simulink model "HybridControllerD3D3"  (Simulink 7.4)
settings: Solver=FixedStepDiscrete  StartTime=0.0  StopTime=inf  FixedStep=samplePeriod  RelTol=1e-3  AbsTol=1e-6
PreLoadFcn:
  | initializeSimulation;
InitFcn:
  | clear('all');
  | initializeSimulation;
undefined symbols (not defined in the file or in its folder): damperA, damperB, damperC, damperCanon, DiscIntNeverNeededParam, flowCanon, forceCanon, frictionA, frictionB, frictionC, gasConstant, HybridCtrlParameters, lengthCanon, massA, massB, massC, massCanon, maxDisplA, maxDisplB, maxDisplC, maxOilVolume, maxVelocA, maxVelocB, maxVelocC, minDisplA, minDisplB, minDisplC, minVelocA, minVelocB, minVelocC, nAct, nAdcU, nDinp, nDout, nDucU, nEncU, precharge, pumpFlow, returnPress, staticForceA, staticForceB, staticForceC, supplyPress, velocCanon, volume, volumeCanon, yieldDisplA, yieldDisplB, yieldDisplC
libraries: simulink x2
(part 1 of 3)
settings Model: Creator=Andreas Schellenberg  LastModifiedBy=Andreas  ExtModeTrigMode=oneshot  ExtModeArmWhenConnect=off  ExtModeAutoUpdateStatusClock=off
settings DataIOCC: SaveOutput=off  SaveTime=off  SignalLoggingName=sigsOut
settings OptimizationCC: EnforceIntegerDowncast=off  InitFltsAndDblsToZero=on
settings DebuggingCC: SaveWithParameterizedLinksMsg=none  CheckSSInitialOutputMsg=off  SolverPrmCheckMsg=none  MultiTaskDSMMsg=warning  MultiTaskCondExecSysMsg=none  StrictBusMsg=None
settings HardwareCC: TargetUnknown=on
settings SFSimCC: SimCustomHeaderCode="#include \"PredictorCorrector.h\""  SimUserSources=PredictorCorrector.c
settings RTWCC: IncludeERTFirstTime=on
settings GRTTargetCC: TargetFcnLib=ansi_tfl_tmw.mat

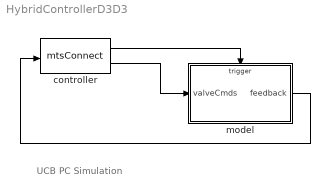
== system HybridControllerD3D3 ==
  note: UCB PC Simulation
  controller : S-Function  FunctionName=mtsConnect  Parameters='127.0.0.1',5002,nUDPInp,nUDPOut  EnableBusSupport=off
  model : Subsystem  TreatAsAtomicUnit=on
  wires:
  model/1(feedback) -> controller/1
  controller/2 -> model/1(valveCmds)
  controller/1 -> model/Trigger

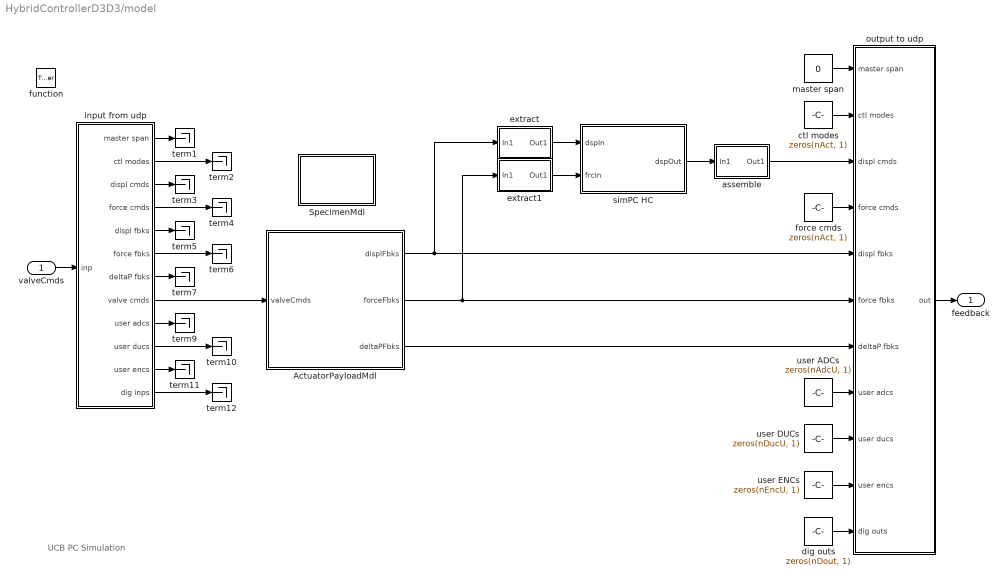
== system HybridControllerD3D3/model ==
  note: UCB PC Simulation
  valveCmds : Inport  OutDataType=sfix(16)  OutScaling=2^0
  function : TriggerPort  TriggerType=function-call
  ActuatorPayloadMdl : Subsystem
  SpecimenMdl : Subsystem
      mask Display: fprintf('Test\nSpecimen');
  assemble : Subsystem  mask(to Actuators){id=1, size=nAct}
      mask prompts: id "Index Vector: id"; size "Vector Size: size"
      mask help: To select to which actuator(s) the signals are going to
      mask Display: disp('Assemble')
  ctl modes : Constant  Value=zeros(nAct, 1)  OutDataType=sfix(16)  OutScaling=2^0
  dig outs : Constant  Value=zeros(nDout, 1)  OutDataTypeMode=uint32  OutDataType=sfix(16)  OutScaling=2^0  OutDataTypeStr=uint32
  extract : Subsystem  mask(from Actuators){id=1, size=nAct}
      mask prompts: id "Index Vector: id"; size "Vector Size: size"
      mask help: To select from which actuator(s) the signals are coming from
      mask Display: disp('Extract')
  extract1 : Subsystem  mask(from Actuators){id=1, size=nAct}
      mask prompts: id "Index Vector: id"; size "Vector Size: size"
      mask help: To select from which actuator(s) the signals are coming from
      mask Display: disp('Extract')
  force cmds : Constant  Value=zeros(nAct, 1)  OutDataType=sfix(16)  OutScaling=2^0
  input from udp : Subsystem
  master span : Constant  Value=0  OutDataType=sfix(16)  OutScaling=2^0
  output to udp : Subsystem
  simPC HC : Subsystem  mask(Hybrid Controller: D3/D3){nAct=1, dtInt=HybridCtrlParameters.dtInt, dtSim=HybridCtrlParameters.dtSim, dtCon=HybridCtrlParameters.dtCon, N=HybridCtrlParameters.N, iDelay=HybridCtrlParameters.iDelay}
      mask prompts: nAct "Number of Actuators: nAct"; dtInt "Integration time step: dtInt"; dtSim "Simulation time step: dtSim"; dtCon "Controller time step: dtCon"; N "Maximum number of substeps: N"; iDelay "Number of delay steps: iDelay"
      mask help: Hybrid Controller using C0-continuous cubic Lagrange interpolation for prediction and correction
      mask Display: disp('simPC Target\nHybrid Controller\n(D3/D3)')
  term{1..7,9..12} (11 alike) : Terminator
  user ADCs : Constant  Value=zeros(nAdcU, 1)  OutDataType=sfix(16)  OutScaling=2^0
  user DUCs : Constant  Value=zeros(nDucU, 1)  OutDataType=sfix(16)  OutScaling=2^0
  user ENCs : Constant  Value=zeros(nEncU, 1)  OutDataType=sfix(16)  OutScaling=2^0
  feedback : Outport  OutDataType=sfix(16)  OutScaling=2^0
  wires:
  input from udp/3(displ cmds) -> term3/1
  input from udp/1(master span) -> term1/1
  input from udp/6(force fbks) -> term6/1
  input from udp/10(user ducs) -> term10/1
  input from udp/12(dig inps) -> term12/1
  input from udp/2(ctl modes) -> term2/1
  input from udp/4(force cmds) -> term4/1
  input from udp/5(displ fbks) -> term5/1
  input from udp/7(deltaP fbks) -> term7/1
  input from udp/9(user adcs) -> term9/1
  input from udp/11(user encs) -> term11/1
  valveCmds/1 -> input from udp/1(inp)
  master span/1 -> output to udp/1(master span)
  ctl modes/1 -> output to udp/2(ctl modes)
  assemble/1(Out1) -> output to udp/3(displ cmds)
  force cmds/1 -> output to udp/4(force cmds)
  user ADCs/1 -> output to udp/8(user adcs)
  user DUCs/1 -> output to udp/9(user ducs)
  user ENCs/1 -> output to udp/10(user encs)
  dig outs/1 -> output to udp/11(dig outs)
  output to udp/1(out) -> feedback/1
  ActuatorPayloadMdl/1(displFbks) -> output to udp/5(displ fbks), extract/1(In1)
  ActuatorPayloadMdl/2(forceFbks) -> output to udp/6(force fbks), extract1/1(In1)
  ActuatorPayloadMdl/3(deltaPFbks) -> output to udp/7(deltaP fbks)
  input from udp/8(valve cmds) -> ActuatorPayloadMdl/1(valveCmds)
  extract1/1(Out1) -> simPC HC/2(frcIn)
  extract/1(Out1) -> simPC HC/1(dspIn)
  simPC HC/1(dspOut) -> assemble/1(In1)

== system HybridControllerD3D3/model/ActuatorPayloadMdl ==
  valveCmds : Inport  OutDataType=sfix(16)  OutScaling=2^0
  Demux : Demux  Outputs=nAct
  Mux : Mux  Inputs=nAct
  Mux1 : Mux  Inputs=nAct
  Mux2 : Mux  Inputs=nAct
  Sum : Sum  Inputs=++++++++  OutDataType=sfix(16)  OutScaling=2^0  SaturateOnIntegerOverflow=on
  accumulators : Subsystem
  dynamic long channel #1 : Subsystem
  dynamic long channel #2 : Subsystem
  dynamic short channel #1 : Subsystem
  dynamic short channel #2 : Subsystem
  static channel #1 : Subsystem
  static channel #2 : Subsystem
  static channel #3 : Subsystem
  static channel #4 : Subsystem
  displFbks : Outport  OutDataType=sfix(16)  OutScaling=2^0
  forceFbks : Outport  Port=2  OutDataType=sfix(16)  OutScaling=2^0
  deltaPFbks : Outport  Port=3  OutDataType=sfix(16)  OutScaling=2^0
  wires:
  Demux/1 -> dynamic short channel #1/1(valve cmd)
  Demux/3 -> dynamic long channel #1/1(valve cmd)
  Demux/2 -> dynamic short channel #2/1(valve cmd)
  dynamic short channel #1/4(flow) -> Sum/1
  dynamic short channel #2/4(flow) -> Sum/2
  dynamic long channel #1/4(flow) -> Sum/3
  Sum/1 -> accumulators/1(flow)
  Demux/4 -> dynamic long channel #2/1(valve cmd)
  Demux/5 -> static channel #1/1(valve cmd)
  Demux/6 -> static channel #2/1(valve cmd)
  Demux/7 -> static channel #3/1(valve cmd)
  Demux/8 -> static channel #4/1(valve cmd)
  dynamic long channel #2/4(flow) -> Sum/4
  static channel #1/4(flow) -> Sum/5
  static channel #2/4(flow) -> Sum/6
  static channel #3/4(flow) -> Sum/7
  static channel #4/4(flow) -> Sum/8
  accumulators/1(press) -> static channel #4/2(spl press), static channel #3/2(spl press), static channel #2/2(spl press), static channel #1/2(spl press), dynamic long channel #2/2(spl press), dynamic long channel #1/2(spl press), dynamic short channel #2/2(spl press), dynamic short channel #1/2(spl press)
  dynamic short channel #1/1(displ) -> Mux/1
  dynamic short channel #2/1(displ) -> Mux/2
  dynamic long channel #1/1(displ) -> Mux/3
  dynamic long channel #2/1(displ) -> Mux/4
  static channel #1/1(displ) -> Mux/5
  static channel #2/1(displ) -> Mux/6
  static channel #3/1(displ) -> Mux/7
  static channel #4/1(displ) -> Mux/8
  dynamic short channel #1/2(force) -> Mux1/1
  dynamic short channel #2/2(force) -> Mux1/2
  dynamic long channel #1/2(force) -> Mux1/3
  dynamic long channel #2/2(force) -> Mux1/4
  static channel #1/2(force) -> Mux1/5
  static channel #2/2(force) -> Mux1/6
  static channel #3/2(force) -> Mux1/7
  static channel #4/2(force) -> Mux1/8
  dynamic short channel #1/3(dpforce) -> Mux2/1
  dynamic short channel #2/3(dpforce) -> Mux2/2
  dynamic long channel #1/3(dpforce) -> Mux2/3
  dynamic long channel #2/3(dpforce) -> Mux2/4
  static channel #1/3(dpforce) -> Mux2/5
  static channel #2/3(dpforce) -> Mux2/6
  static channel #3/3(dpforce) -> Mux2/7
  static channel #4/3(dpforce) -> Mux2/8
  valveCmds/1 -> Demux/1
  Mux/1 -> displFbks/1
  Mux1/1 -> forceFbks/1
  Mux2/1 -> deltaPFbks/1

== system HybridControllerD3D3/model/SpecimenMdl ==
  Scope3 : Scope
      settings: TimeRange=250  YMin=-2  YMax=2  SaveName=ScopeData2
  Specimen #1 : S-Function  FunctionName=SFun_SimFEAdapter  Parameters=ipAddr,ipPort,dataSize  EnableBusSupport=off  mask(GenericClient Element){ipAddr=127.0.0.1, ipPort=44000, dataSize=256}
      mask prompts: ipAddr "IP Address of Adapter Element"; ipPort "IP Port Number of Adapter Element"; dataSize "Size of Data Arrays"
      mask Display: disp('SimFE\nAdapter');
  Terminator : Terminator
  assemble1 : Subsystem  mask(to Actuators){id=1, size=nAct}
      mask prompts: id "Index Vector: id"; size "Vector Size: size"
      mask help: To select to which actuator(s) the signals are going to
      mask Display: disp('Assemble')
  assemble2 : Subsystem  mask(to Actuators){id=1, size=nAct}
      mask prompts: id "Index Vector: id"; size "Vector Size: size"
      mask help: To select to which actuator(s) the signals are going to
      mask Display: disp('Assemble')
  extract2 : Subsystem  mask(from Actuators){id=1, size=nAct}
      mask prompts: id "Index Vector: id"; size "Vector Size: size"
      mask help: To select from which actuator(s) the signals are coming from
      mask Display: disp('Extract')
  from Actuators : Subsystem
  to LoadCells : Subsystem
  wires:
  from Actuators/1(ctrlDisp) -> extract2/1(In1)
  extract2/1(Out1) -> Specimen #1/1
  Specimen #1/1 -> assemble2/1(In1)
  Specimen #1/2 -> assemble1/1(In1), Scope3/1
  assemble2/1(Out1) -> Terminator/1
  assemble1/1(Out1) -> to LoadCells/1(daqForce)

== system HybridControllerD3D3/model/assemble ==
  In1 : Inport  OutDataType=sfix(16)  OutScaling=2^0
  Assignment : Assignment  OutputInitialize=Specify size for each dimension in table  IndexOptions=Index vector (port)  Indices=1  OutputSizes=nAct
  Constant : Constant  Value=id  OutDataType=sfix(16)  OutScaling=2^0
  Out1 : Outport  OutDataType=sfix(16)  OutScaling=2^0
  wires:
  Constant/1 -> Assignment/2
  Assignment/1 -> Out1/1
  In1/1 -> Assignment/1

== system HybridControllerD3D3/model/extract ==
  In1 : Inport  OutDataType=sfix(16)  OutScaling=2^0
  Selector : Selector  InputPortWidth=size  IndexOptions=Index vector (dialog)  Indices=id  OutputSizes=1
  Out1 : Outport  OutDataType=sfix(16)  OutScaling=2^0
  wires:
  Selector/1 -> Out1/1
  In1/1 -> Selector/1

== system HybridControllerD3D3/model/extract1 ==
  In1 : Inport  OutDataType=sfix(16)  OutScaling=2^0
  Selector : Selector  InputPortWidth=size  IndexOptions=Index vector (dialog)  Indices=id  OutputSizes=1
  Out1 : Outport  OutDataType=sfix(16)  OutScaling=2^0
  wires:
  Selector/1 -> Out1/1
  In1/1 -> Selector/1

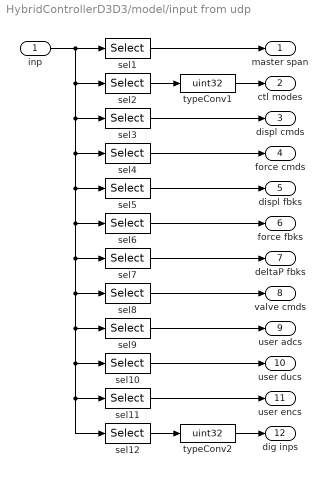
== system HybridControllerD3D3/model/input from udp ==
  inp : Inport  OutDataType=sfix(16)  OutScaling=2^0
  sel1 : Selector  InputPortWidth=nUDPOut  IndexOptions=Index vector (dialog)  Indices=[0]+1  OutputSizes=1
  sel10 : Selector  InputPortWidth=nUDPOut  IndexOptions=Index vector (dialog)  Indices=[1:nDucU]+1+7*nAct+nAdcU  OutputSizes=1
  sel11 : Selector  InputPortWidth=nUDPOut  IndexOptions=Index vector (dialog)  Indices=[1:nEncU]+1+7*nAct+nAdcU+nDucU  OutputSizes=1
  sel12 : Selector  InputPortWidth=nUDPOut  IndexOptions=Index vector (dialog)  Indices=[1:nDinp]+1+7*nAct+nAdcU+nDucU+nEncU  OutputSizes=1
  sel2 : Selector  InputPortWidth=nUDPOut  IndexOptions=Index vector (dialog)  Indices=[1:nAct]+1+0*nAct  OutputSizes=1
  sel3 : Selector  InputPortWidth=nUDPOut  IndexOptions=Index vector (dialog)  Indices=[1:nAct]+1+1*nAct  OutputSizes=1
  sel4 : Selector  InputPortWidth=nUDPOut  IndexOptions=Index vector (dialog)  Indices=[1:nAct]+1+2*nAct  OutputSizes=1
  sel5 : Selector  InputPortWidth=nUDPOut  IndexOptions=Index vector (dialog)  Indices=[1:nAct]+1+3*nAct  OutputSizes=1
  sel6 : Selector  InputPortWidth=nUDPOut  IndexOptions=Index vector (dialog)  Indices=[1:nAct]+1+4*nAct  OutputSizes=1
  sel7 : Selector  InputPortWidth=nUDPOut  IndexOptions=Index vector (dialog)  Indices=[1:nAct]+1+5*nAct  OutputSizes=1
  sel8 : Selector  InputPortWidth=nUDPOut  IndexOptions=Index vector (dialog)  Indices=[1:nAct]+1+6*nAct  OutputSizes=1
  sel9 : Selector  InputPortWidth=nUDPOut  IndexOptions=Index vector (dialog)  Indices=[1:nAdcU]+1+7*nAct  OutputSizes=1
  typeConv1 : DataTypeConversion  OutDataTypeMode=uint32  OutDataType=sfix(16)  OutScaling=2^0  OutDataTypeStr=uint32  SaturateOnIntegerOverflow=on  RndMeth=Zero
  typeConv2 : DataTypeConversion  OutDataTypeMode=uint32  OutDataType=sfix(16)  OutScaling=2^0  OutDataTypeStr=uint32  SaturateOnIntegerOverflow=on  RndMeth=Zero
  master span : Outport  OutDataType=sfix(16)  OutScaling=2^0
  ctl modes : Outport  Port=2  OutDataType=sfix(16)  OutScaling=2^0
  displ cmds : Outport  Port=3  OutDataType=sfix(16)  OutScaling=2^0
  force cmds : Outport  Port=4  OutDataType=sfix(16)  OutScaling=2^0
  displ fbks : Outport  Port=5  OutDataType=sfix(16)  OutScaling=2^0
  force fbks : Outport  Port=6  OutDataType=sfix(16)  OutScaling=2^0
  deltaP fbks : Outport  Port=7  OutDataType=sfix(16)  OutScaling=2^0
  valve cmds : Outport  Port=8  OutDataType=sfix(16)  OutScaling=2^0
  user adcs : Outport  Port=9  OutDataType=sfix(16)  OutScaling=2^0
  user ducs : Outport  Port=10  OutDataType=sfix(16)  OutScaling=2^0
  user encs : Outport  Port=11  OutDataType=sfix(16)  OutScaling=2^0
  dig inps : Outport  Port=12  OutDataType=sfix(16)  OutScaling=2^0
  wires:
  sel1/1 -> master span/1
  sel2/1 -> typeConv1/1
  sel3/1 -> displ cmds/1
  sel4/1 -> force cmds/1
  sel5/1 -> displ fbks/1
  sel6/1 -> force fbks/1
  sel7/1 -> deltaP fbks/1
  sel8/1 -> valve cmds/1
  sel9/1 -> user adcs/1
  sel10/1 -> user ducs/1
  sel11/1 -> user encs/1
  sel12/1 -> typeConv2/1
  inp/1 -> sel1/1, sel2/1, sel3/1, sel11/1, sel12/1, sel10/1, sel9/1, sel8/1, sel7/1, sel6/1, sel5/1, sel4/1
  typeConv1/1 -> ctl modes/1
  typeConv2/1 -> dig inps/1

== system HybridControllerD3D3/model/output to udp ==
  master span : Inport  OutDataType=sfix(16)  OutScaling=2^0
  ctl modes : Inport  Port=2  OutDataType=sfix(16)  OutScaling=2^0
  displ cmds : Inport  Port=3  OutDataType=sfix(16)  OutScaling=2^0
  force cmds : Inport  Port=4  OutDataType=sfix(16)  OutScaling=2^0
  displ fbks : Inport  Port=5  OutDataType=sfix(16)  OutScaling=2^0
  force fbks : Inport  Port=6  OutDataType=sfix(16)  OutScaling=2^0
  deltaP fbks : Inport  Port=7  OutDataType=sfix(16)  OutScaling=2^0
  user adcs : Inport  Port=8  OutDataType=sfix(16)  OutScaling=2^0
  user ducs : Inport  Port=9  OutDataType=sfix(16)  OutScaling=2^0
  user encs : Inport  Port=10  OutDataType=sfix(16)  OutScaling=2^0
  dig outs : Inport  Port=11  OutDataType=sfix(16)  OutScaling=2^0
  Mux : Mux  Inputs=11
  typeConv1 : DataTypeConversion  OutDataTypeMode=double  OutDataType=sfix(16)  OutScaling=2^0  OutDataTypeStr=double  SaturateOnIntegerOverflow=on  RndMeth=Zero
  typeConv2 : DataTypeConversion  OutDataTypeMode=double  OutDataType=sfix(16)  OutScaling=2^0  OutDataTypeStr=double  SaturateOnIntegerOverflow=on  RndMeth=Zero
  out : Outport  OutDataType=sfix(16)  OutScaling=2^0
  wires:
  typeConv2/1 -> Mux/11
  dig outs/1 -> typeConv2/1
  user encs/1 -> Mux/10
  user ducs/1 -> Mux/9
  user adcs/1 -> Mux/8
  deltaP fbks/1 -> Mux/7
  force fbks/1 -> Mux/6
  displ fbks/1 -> Mux/5
  force cmds/1 -> Mux/4
  master span/1 -> Mux/1
  displ cmds/1 -> Mux/3
  ctl modes/1 -> typeConv1/1
  Mux/1 -> out/1
  typeConv1/1 -> Mux/2

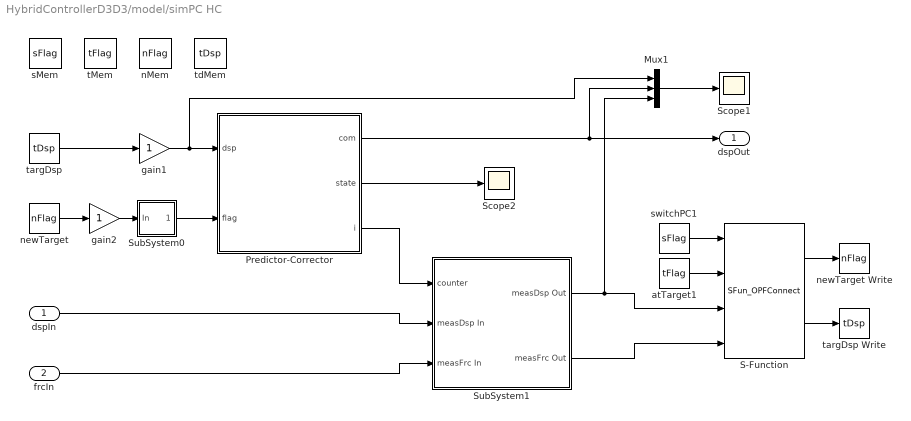
== system HybridControllerD3D3/model/simPC HC ==
  dspIn : Inport  OutDataType=sfix(16)  OutScaling=2^0
  frcIn : Inport  Port=2  OutDataType=sfix(16)  OutScaling=2^0
  Mux1 : Mux  Inputs=3
  Predictor-Corrector : Stateflow chart
  S-Function : S-Function  FunctionName=SFun_OPFConnect  Parameters=ipPort  EnableBusSupport=off  mask(OpenFresco Connect){ipPort=8090}
      mask prompts: ipPort "IP Port Number of Server"
      mask Display: disp('OpenFresco\nConnect');
  Scope1 : Scope
      settings: TimeRange=250  YMin=-2  YMax=2.5  SaveName=ScopeData3
  Scope2 : Scope
      settings: TimeRange=250  YMin=0  YMax=2  SaveName=ScopeData2
  SubSystem0 : Subsystem
  SubSystem1 : Subsystem
  atTarget1 : DataStoreRead  DataStoreName=tFlag  SampleTime=-1
  gain1 : Gain  ParameterDataType=sfix(16)  ParameterScaling=2^0  OutDataType=sfix(16)  OutScaling=2^0
  gain2 : Gain  ParameterDataType=sfix(16)  ParameterScaling=2^0  OutDataType=sfix(16)  OutScaling=2^0
  nMem : DataStoreMemory  DataStoreName=nFlag  DataType=double  OutDataType=sfix(16)  OutScaling=2^0  OutDataTypeStr=double
  newTarget : DataStoreRead  DataStoreName=nFlag  SampleTime=-1
  newTarget Write : DataStoreWrite  DataStoreName=nFlag  SampleTime=-1
  sMem : DataStoreMemory  DataStoreName=sFlag  DataType=double  OutDataType=sfix(16)  OutScaling=2^0  OutDataTypeStr=double
  switchPC1 : DataStoreRead  DataStoreName=sFlag  SampleTime=-1
  tMem : DataStoreMemory  DataStoreName=tFlag  DataType=double  OutDataType=sfix(16)  OutScaling=2^0  OutDataTypeStr=double
  targDsp : DataStoreRead  DataStoreName=tDsp  SampleTime=-1
  targDsp Write : DataStoreWrite  DataStoreName=tDsp  SampleTime=-1
  tdMem : DataStoreMemory  DataStoreName=tDsp  DataType=double  OutDataType=sfix(16)  OutScaling=2^0  OutDataTypeStr=double
  dspOut : Outport  OutDataType=sfix(16)  OutScaling=2^0
  wires:
  frcIn/1 -> SubSystem1/3(measFrc In)
  dspIn/1 -> SubSystem1/2(measDsp In)
  SubSystem1/2(measFrc Out) -> S-Function/4
  SubSystem1/1(measDsp Out) -> Mux1/3, S-Function/3
  Predictor-Corrector/3(i) -> SubSystem1/1(counter)
  Predictor-Corrector/2(state) -> Scope2/1
  Predictor-Corrector/1(com) -> dspOut/1, Mux1/2
  SubSystem0/1(Out) -> Predictor-Corrector/2(flag)
  newTarget/1 -> gain2/1
  gain2/1 -> SubSystem0/1(In)
  targDsp/1 -> gain1/1
  gain1/1 -> Predictor-Corrector/1(dsp), Mux1/1
  Mux1/1 -> Scope1/1
  switchPC1/1 -> S-Function/1
  atTarget1/1 -> S-Function/2
  S-Function/1 -> newTarget Write/1
  S-Function/2 -> targDsp Write/1

== system HybridControllerD3D3/model/ActuatorPayloadMdl/accumulators ==
  flow : Inport  OutDataType=sfix(16)  OutScaling=2^0
  Sum : Sum  Inputs=+-|  OutDataType=sfix(16)  OutScaling=2^0  SaturateOnIntegerOverflow=on  InputSameDT=on  OutDataTypeStr=Inherit: Same as first input
  Sum1 : Sum  Inputs=+-|  OutDataType=sfix(16)  OutScaling=2^0  SaturateOnIntegerOverflow=on  InputSameDT=on  OutDataTypeStr=Inherit: Same as first input
  bottle volume : Constant  Value=volume*volumeCanon  OutDataType=sfix(16)  OutScaling=2^0
  flowCanon : Gain  Gain=flowCanon  ParameterDataType=sfix(16)  ParameterScaling=2^0  OutDataType=sfix(16)  OutScaling=2^0  SaturateOnIntegerOverflow=on  OutDataTypeStr=Inherit: Same as input  ParamDataTypeStr=Inherit: Same as input
  gas constant : Constant  Value=gasConstant  OutDataType=sfix(16)  OutScaling=2^0
  initial condition : UnitDelay  X0=supplyPress  SampleTime=-1
  integrator : DiscreteIntegrator  InitialCondition=maxOilVolume*volumeCanon  SampleTime=-1  OutDataType=sfix(16)  OutScaling=2^0  LimitOutput=on  UpperSaturationLimit=maxOilVolume*volumeCanon  LowerSaturationLimit=0  ICPrevOutput=DiscIntNeverNeededParam  ICPrevScaledInput=DiscIntNeverNeededParam
  power : Math  Operator=pow  OutDataType=sfix(16)  OutScaling=2^0  SaturateOnIntegerOverflow=on
  precharge : Gain  Gain=precharge  ParameterDataType=sfix(16)  ParameterScaling=2^0  OutDataType=sfix(16)  OutScaling=2^0  SaturateOnIntegerOverflow=on  OutDataTypeStr=Inherit: Same as input  ParamDataTypeStr=Inherit: Same as input
  pump flow : Constant  Value=pumpFlow  OutDataType=sfix(16)  OutScaling=2^0
  quotient : Product  Inputs=*/  OutDataType=sfix(16)  OutScaling=2^0  SaturateOnIntegerOverflow=on  InputSameDT=on  OutDataTypeStr=Inherit: Same as first input
  press : Outport  OutDataType=sfix(16)  OutScaling=2^0
  wires:
  initial condition/1 -> press/1
  flowCanon/1 -> integrator/1
  flow/1 -> Sum/2
  integrator/1 -> Sum1/2  "current oil volume"
  quotient/1 -> power/1
  Sum1/1 -> quotient/2  "current gas volume"
  precharge/1 -> initial condition/1
  power/1 -> precharge/1
  gas constant/1 -> power/2
  bottle volume/1 -> quotient/1, Sum1/1
  Sum/1 -> flowCanon/1
  pump flow/1 -> Sum/1

== system HybridControllerD3D3/model/ActuatorPayloadMdl/dynamic long channel #1 ==
  valve cmd : Inport  OutDataType=sfix(16)  OutScaling=2^0
  spl press : Inport  Port=2  OutDataType=sfix(16)  OutScaling=2^0
  actuator/valve  model : Subsystem
      mask Type: Inverse Actuator
  payload : Subsystem
  return pressure : Constant  Value=returnPress  OutDataType=sfix(16)  OutScaling=2^0
  displ : Outport  OutDataType=sfix(16)  OutScaling=2^0
  force : Outport  Port=2  OutDataType=sfix(16)  OutScaling=2^0
  dpforce : Outport  Port=3  OutDataType=sfix(16)  OutScaling=2^0
  flow : Outport  Port=4  OutDataType=sfix(16)  OutScaling=2^0
  wires:
  payload/2(veloc) -> actuator/valve  model/3(veloc)
  payload/1(displ) -> displ/1, actuator/valve  model/2(displ)
  valve cmd/1 -> actuator/valve  model/1(cmd)
  return pressure/1 -> actuator/valve  model/5(rtn press)
  spl press/1 -> actuator/valve  model/4(spl press)
  actuator/valve  model/2(flow) -> flow/1
  actuator/valve  model/1(force) -> force/1, dpforce/1, payload/1(force)

== system HybridControllerD3D3/model/ActuatorPayloadMdl/dynamic long channel #2 ==
  valve cmd : Inport  OutDataType=sfix(16)  OutScaling=2^0
  spl press : Inport  Port=2  OutDataType=sfix(16)  OutScaling=2^0
  actuator/valve  model : Subsystem
      mask Type: Inverse Actuator
  payload : Subsystem
  return pressure : Constant  Value=returnPress  OutDataType=sfix(16)  OutScaling=2^0
  displ : Outport  OutDataType=sfix(16)  OutScaling=2^0
  force : Outport  Port=2  OutDataType=sfix(16)  OutScaling=2^0
  dpforce : Outport  Port=3  OutDataType=sfix(16)  OutScaling=2^0
  flow : Outport  Port=4  OutDataType=sfix(16)  OutScaling=2^0
  wires:
  actuator/valve  model/1(force) -> dpforce/1, force/1, payload/1(force)
  actuator/valve  model/2(flow) -> flow/1
  spl press/1 -> actuator/valve  model/4(spl press)
  return pressure/1 -> actuator/valve  model/5(rtn press)
  valve cmd/1 -> actuator/valve  model/1(cmd)
  payload/1(displ) -> actuator/valve  model/2(displ), displ/1
  payload/2(veloc) -> actuator/valve  model/3(veloc)

== system HybridControllerD3D3/model/ActuatorPayloadMdl/dynamic short channel #1 ==
  valve cmd : Inport  OutDataType=sfix(16)  OutScaling=2^0
  spl press : Inport  Port=2  OutDataType=sfix(16)  OutScaling=2^0
  actuator/valve  model : Subsystem
      mask Type: Inverse Actuator
  payload : Subsystem
  return pressure : Constant  Value=returnPress  OutDataType=sfix(16)  OutScaling=2^0
  displ : Outport  OutDataType=sfix(16)  OutScaling=2^0
  force : Outport  Port=2  OutDataType=sfix(16)  OutScaling=2^0
  dpforce : Outport  Port=3  OutDataType=sfix(16)  OutScaling=2^0
  flow : Outport  Port=4  OutDataType=sfix(16)  OutScaling=2^0
  wires:
  actuator/valve  model/1(force) -> dpforce/1, force/1, payload/1(force)
  actuator/valve  model/2(flow) -> flow/1
  spl press/1 -> actuator/valve  model/4(spl press)
  return pressure/1 -> actuator/valve  model/5(rtn press)
  valve cmd/1 -> actuator/valve  model/1(cmd)
  payload/1(displ) -> actuator/valve  model/2(displ), displ/1
  payload/2(veloc) -> actuator/valve  model/3(veloc)

== system HybridControllerD3D3/model/ActuatorPayloadMdl/dynamic short channel #2 ==
  valve cmd : Inport  OutDataType=sfix(16)  OutScaling=2^0
  spl press : Inport  Port=2  OutDataType=sfix(16)  OutScaling=2^0
  actuator/valve  model : Subsystem
      mask Type: Inverse Actuator
  payload : Subsystem
  return pressure : Constant  Value=returnPress  OutDataType=sfix(16)  OutScaling=2^0
  displ : Outport  OutDataType=sfix(16)  OutScaling=2^0
  force : Outport  Port=2  OutDataType=sfix(16)  OutScaling=2^0
  dpforce : Outport  Port=3  OutDataType=sfix(16)  OutScaling=2^0
  flow : Outport  Port=4  OutDataType=sfix(16)  OutScaling=2^0
  wires:
  actuator/valve  model/1(force) -> dpforce/1, force/1, payload/1(force)
  actuator/valve  model/2(flow) -> flow/1
  spl press/1 -> actuator/valve  model/4(spl press)
  return pressure/1 -> actuator/valve  model/5(rtn press)
  valve cmd/1 -> actuator/valve  model/1(cmd)
  payload/1(displ) -> actuator/valve  model/2(displ), displ/1
  payload/2(veloc) -> actuator/valve  model/3(veloc)

== system HybridControllerD3D3/model/ActuatorPayloadMdl/static channel #1 ==
  valve cmd : Inport  OutDataType=sfix(16)  OutScaling=2^0
  spl press : Inport  Port=2  OutDataType=sfix(16)  OutScaling=2^0
  actuator/valve  model : Subsystem
      mask Type: Inverse Actuator
  payload : Subsystem
  return pressure : Constant  Value=returnPress  OutDataType=sfix(16)  OutScaling=2^0
  displ : Outport  OutDataType=sfix(16)  OutScaling=2^0
  force : Outport  Port=2  OutDataType=sfix(16)  OutScaling=2^0
  dpforce : Outport  Port=3  OutDataType=sfix(16)  OutScaling=2^0
  flow : Outport  Port=4  OutDataType=sfix(16)  OutScaling=2^0
  wires:
  payload/2(veloc) -> actuator/valve  model/3(veloc)
  payload/1(displ) -> displ/1, actuator/valve  model/2(displ)
  valve cmd/1 -> actuator/valve  model/1(cmd)
  return pressure/1 -> actuator/valve  model/5(rtn press)
  spl press/1 -> actuator/valve  model/4(spl press)
  actuator/valve  model/2(flow) -> flow/1
  actuator/valve  model/1(force) -> force/1, dpforce/1, payload/1(force)

== system HybridControllerD3D3/model/ActuatorPayloadMdl/static channel #2 ==
  valve cmd : Inport  OutDataType=sfix(16)  OutScaling=2^0
  spl press : Inport  Port=2  OutDataType=sfix(16)  OutScaling=2^0
  actuator/valve  model : Subsystem
      mask Type: Inverse Actuator
  payload : Subsystem
  return pressure : Constant  Value=returnPress  OutDataType=sfix(16)  OutScaling=2^0
  displ : Outport  OutDataType=sfix(16)  OutScaling=2^0
  force : Outport  Port=2  OutDataType=sfix(16)  OutScaling=2^0
  dpforce : Outport  Port=3  OutDataType=sfix(16)  OutScaling=2^0
  flow : Outport  Port=4  OutDataType=sfix(16)  OutScaling=2^0
  wires:
  actuator/valve  model/1(force) -> dpforce/1, force/1, payload/1(force)
  actuator/valve  model/2(flow) -> flow/1
  spl press/1 -> actuator/valve  model/4(spl press)
  return pressure/1 -> actuator/valve  model/5(rtn press)
  valve cmd/1 -> actuator/valve  model/1(cmd)
  payload/1(displ) -> actuator/valve  model/2(displ), displ/1
  payload/2(veloc) -> actuator/valve  model/3(veloc)

== system HybridControllerD3D3/model/ActuatorPayloadMdl/static channel #3 ==
  valve cmd : Inport  OutDataType=sfix(16)  OutScaling=2^0
  spl press : Inport  Port=2  OutDataType=sfix(16)  OutScaling=2^0
  actuator/valve  model : Subsystem
      mask Type: Inverse Actuator
  payload : Subsystem
  return pressure : Constant  Value=returnPress  OutDataType=sfix(16)  OutScaling=2^0
  displ : Outport  OutDataType=sfix(16)  OutScaling=2^0
  force : Outport  Port=2  OutDataType=sfix(16)  OutScaling=2^0
  dpforce : Outport  Port=3  OutDataType=sfix(16)  OutScaling=2^0
  flow : Outport  Port=4  OutDataType=sfix(16)  OutScaling=2^0
  wires:
  payload/2(veloc) -> actuator/valve  model/3(veloc)
  payload/1(displ) -> displ/1, actuator/valve  model/2(displ)
  valve cmd/1 -> actuator/valve  model/1(cmd)
  return pressure/1 -> actuator/valve  model/5(rtn press)
  spl press/1 -> actuator/valve  model/4(spl press)
  actuator/valve  model/2(flow) -> flow/1
  actuator/valve  model/1(force) -> force/1, dpforce/1, payload/1(force)

== system HybridControllerD3D3/model/ActuatorPayloadMdl/static channel #4 ==
  valve cmd : Inport  OutDataType=sfix(16)  OutScaling=2^0
  spl press : Inport  Port=2  OutDataType=sfix(16)  OutScaling=2^0
  actuator/valve  model : Subsystem
      mask Type: Inverse Actuator
  payload : Subsystem
  return pressure : Constant  Value=returnPress  OutDataType=sfix(16)  OutScaling=2^0
  displ : Outport  OutDataType=sfix(16)  OutScaling=2^0
  force : Outport  Port=2  OutDataType=sfix(16)  OutScaling=2^0
  dpforce : Outport  Port=3  OutDataType=sfix(16)  OutScaling=2^0
  flow : Outport  Port=4  OutDataType=sfix(16)  OutScaling=2^0
  wires:
  actuator/valve  model/1(force) -> dpforce/1, force/1, payload/1(force)
  actuator/valve  model/2(flow) -> flow/1
  spl press/1 -> actuator/valve  model/4(spl press)
  return pressure/1 -> actuator/valve  model/5(rtn press)
  valve cmd/1 -> actuator/valve  model/1(cmd)
  payload/1(displ) -> actuator/valve  model/2(displ), displ/1
  payload/2(veloc) -> actuator/valve  model/3(veloc)

== system HybridControllerD3D3/model/SpecimenMdl/assemble1 ==
  In1 : Inport  OutDataType=sfix(16)  OutScaling=2^0
  Assignment : Assignment  OutputInitialize=Specify size for each dimension in table  IndexOptions=Index vector (port)  Indices=1  OutputSizes=nAct
  Constant : Constant  Value=id  OutDataType=sfix(16)  OutScaling=2^0
  Out1 : Outport  OutDataType=sfix(16)  OutScaling=2^0
  wires:
  Constant/1 -> Assignment/2
  Assignment/1 -> Out1/1
  In1/1 -> Assignment/1

== system HybridControllerD3D3/model/SpecimenMdl/assemble2 ==
  In1 : Inport  OutDataType=sfix(16)  OutScaling=2^0
  Assignment : Assignment  OutputInitialize=Specify size for each dimension in table  IndexOptions=Index vector (port)  Indices=1  OutputSizes=nAct
  Constant : Constant  Value=id  OutDataType=sfix(16)  OutScaling=2^0
  Out1 : Outport  OutDataType=sfix(16)  OutScaling=2^0
  wires:
  Constant/1 -> Assignment/2
  Assignment/1 -> Out1/1
  In1/1 -> Assignment/1

== system HybridControllerD3D3/model/SpecimenMdl/extract2 ==
  In1 : Inport  OutDataType=sfix(16)  OutScaling=2^0
  Selector : Selector  InputPortWidth=size  IndexOptions=Index vector (dialog)  Indices=id  OutputSizes=1
  Out1 : Outport  OutDataType=sfix(16)  OutScaling=2^0
  wires:
  Selector/1 -> Out1/1
  In1/1 -> Selector/1

== system HybridControllerD3D3/model/SpecimenMdl/from Actuators ==
  Bus Creator : BusCreator  Inputs=8
  ctrlDisp : Outport
  wires:
  [ch1a] -> Bus Creator/1
  [ch2a] -> Bus Creator/2
  [ch3a] -> Bus Creator/3
  [ch4a] -> Bus Creator/4
  [ch5a] -> Bus Creator/5
  [ch6a] -> Bus Creator/6
  [ch7a] -> Bus Creator/7
  [ch8a] -> Bus Creator/8
  Bus Creator/1 -> ctrlDisp/1

== system HybridControllerD3D3/model/SpecimenMdl/to LoadCells ==
  daqForce : Inport
  Demux : Demux  Outputs=8
  tag scope: ch1b=global, ch2b=global, ch3b=global, ch4b=global, ch5b=global, ch6b=global, ch7b=global, ch8b=global
  wires:
  Demux/1 -> [ch1b]
  Demux/2 -> [ch2b]
  Demux/3 -> [ch3b]
  Demux/4 -> [ch4b]
  Demux/5 -> [ch5b]
  Demux/6 -> [ch6b]
  Demux/7 -> [ch7b]
  Demux/8 -> [ch8b]
  daqForce/1 -> Demux/1

== system HybridControllerD3D3/model/simPC HC/SubSystem0 ==
  In : Inport  OutDataType=sfix(16)  OutScaling=2^0
  Detect Fall Nonpositive : simulink/Logic and Bit Operations/Detect Fall Nonpositive  SystemSampleTime=-1  vinit=0
  Detect Rise Positive : simulink/Logic and Bit Operations/Detect Rise Positive  SystemSampleTime=-1  vinit=0
  If Action Subsystem0 : Subsystem  TreatAsAtomicUnit=on
  If Action Subsystem1 : Subsystem  TreatAsAtomicUnit=on
  If0 : If  IfExpression=u1 == 1  ShowElse=off
  If1 : If  IfExpression=u1 == 1  ShowElse=off
  Mux1 : Mux  Inputs=3
  Scope3 : Scope
      settings: TimeRange=250  YMin=0  YMax=1
  atTarget1 : DataStoreRead  DataStoreName=tFlag  SampleTime=-1
  switchPC1 : DataStoreRead  DataStoreName=sFlag  SampleTime=-1
  typeConv : DataTypeConversion  OutDataTypeMode=double  OutDataType=sfix(16)  OutScaling=2^0  OutDataTypeStr=double  SaturateOnIntegerOverflow=on  RndMeth=Zero
  Out : Outport  OutDataType=sfix(16)  OutScaling=2^0
  wires:
  In/1 -> Detect Rise Positive/1, Detect Fall Nonpositive/1, Mux1/1
  Detect Rise Positive/1 -> If0/1, typeConv/1
  Detect Fall Nonpositive/1 -> If1/1
  If1/1 -> If Action Subsystem1/Action
  If0/1 -> If Action Subsystem0/Action
  typeConv/1 -> Out/1
  Mux1/1 -> Scope3/1
  switchPC1/1 -> Mux1/2
  atTarget1/1 -> Mux1/3

== system HybridControllerD3D3/model/simPC HC/SubSystem1 ==
  counter : Inport  OutDataType=sfix(16)  OutScaling=2^0
  measDsp In : Inport  Port=2  OutDataType=sfix(16)  OutScaling=2^0
  measFrc In : Inport  Port=3  OutDataType=sfix(16)  OutScaling=2^0
  Hit  Crossing : HitCross  HitCrossingOffset=iDelay
  SubSystem : Subsystem  TreatAsAtomicUnit=on
  measDsp Out : Outport  OutDataType=sfix(16)  OutScaling=2^0
  measFrc Out : Outport  Port=2  OutDataType=sfix(16)  OutScaling=2^0
  wires:
  SubSystem/2(measFrc Out) -> measFrc Out/1
  measFrc In/1 -> SubSystem/2(measFrc In)
  SubSystem/1(measDsp Out) -> measDsp Out/1
  measDsp In/1 -> SubSystem/1(measDsp In)
  counter/1 -> Hit  Crossing/1
  Hit  Crossing/1 -> SubSystem/Trigger

== system HybridControllerD3D3/model/ActuatorPayloadMdl/dynamic long channel #1/actuator/valve  model ==
  note: Note: "1" and "2" denote actuator
      | cylinders on either side of the
      | actuator piston.  With positive
      | valve drive, oil is ported into
      | cylinder 1, resulting in positive
      | displacement.
  note: Auxiliary diagnostic output vector:
      | 1:   valve opening
      | 2:   C1 pressure
      | 3:   C2 pressure
      | 4:   delta pressure
      | 5:   force
      | 6:   velocity
      | 7:   C1 flow
      | 8:   C2 flow
      | 9:   total flow
      | 10: kinematic flow
      | 11: compressibility flow
      | 12: leakage flow
  note: Parameter vector:
      | 1:   oil bulk modulus (force/displ^2)
      | 2:   servovalve delay (sec)
      | 3:   servovalve overlap
      | 4:   rated pressure (force/displ^2)
      | 5:   rated flow at rated pressure (displ^3/sec)
      | 6:   nominal flow at rated pressure (displ^3/sec)
      | 7:   actuator piston area 1 (displ^2)
      | 8:   actuator piston area 2 (displ^2)
      | 9:   actuator usable stroke 1 (displ)
      | 10: actuator usable stroke 2 (displ)
      | 11: actuator end cushion length 1 (displ)
      | 12: actuator end cushion length 2 (displ)
      | 13: actuator parasitic damping factor
      | 14: cross-chamber leakage factor (flow/press)
      | 15: ratio port openings according to area
      | 16: sample period (sec)
      |
      | Conversion factors used for converting
      | signals from external (user) to internal
      | (canonical) units:
      |
      | 17: displacement
      | 18: velocity
      | 19: force
      | 20: pressure
      | 21: flow
  cmd : Inport  OutDataType=sfix(16)  OutScaling=2^0
  displ : Inport  Port=2  OutDataType=sfix(16)  OutScaling=2^0
  veloc : Inport  Port=3  OutDataType=sfix(16)  OutScaling=2^0
  spl press : Inport  Port=4  OutDataType=sfix(16)  OutScaling=2^0
  rtn press : Inport  Port=5  OutDataType=sfix(16)  OutScaling=2^0
  abs : Abs  SaturateOnIntegerOverflow=on
  actuator : S-Function  FunctionName=actuator  Parameters=actParamsB  EnableBusSupport=off
  total flow sel : Selector  InputPortWidth=12  IndexOptions=Index vector (dialog)  Indices=9  OutputSizes=1
  force : Outport  OutDataType=sfix(16)  OutScaling=2^0
  flow : Outport  Port=2  OutDataType=sfix(16)  OutScaling=2^0
  wires:
  veloc/1 -> actuator/3
  displ/1 -> actuator/2
  actuator/1 -> force/1
  cmd/1 -> actuator/1
  rtn press/1 -> actuator/5
  spl press/1 -> actuator/4
  total flow sel/1 -> abs/1
  actuator/2 -> total flow sel/1
  abs/1 -> flow/1

== system HybridControllerD3D3/model/ActuatorPayloadMdl/dynamic long channel #1/payload ==
  force : Inport  OutDataType=sfix(16)  OutScaling=2^0
  Sum : Sum  Inputs=+----  OutDataType=sfix(16)  OutScaling=2^0  SaturateOnIntegerOverflow=on  InputSameDT=on  OutDataTypeStr=Inherit: Same as first input
  damper : Gain  Gain=damperB*damperCanon  ParameterDataType=sfix(16)  ParameterScaling=2^0  OutDataType=sfix(16)  OutScaling=2^0  SaturateOnIntegerOverflow=on  OutDataTypeStr=Inherit: Same as input  ParamDataTypeStr=Inherit: Same as input
  div : Product  Inputs=*/  OutDataType=sfix(16)  OutScaling=2^0  SaturateOnIntegerOverflow=on  InputSameDT=on  OutDataTypeStr=Inherit: Same as first input
  double integrator : Subsystem
  friction : Subsystem  mask{friction=frictionB*forceCanon, yieldDispl=yieldDisplB*lengthCanon, hysteresis=0}
      mask prompts: friction "Sliding friction"; yieldDispl "Equiv. yield displacement (in)"; hysteresis "Hysteresis constant"
  mass : Constant  Value=massB*massCanon  OutDataType=sfix(16)  OutScaling=2^0
  static force : Constant  Value=staticForceB*forceCanon  OutDataType=sfix(16)  OutScaling=2^0
  term1 : Terminator
  unit dly : UnitDelay  SampleTime=-1
  unit dly1 : UnitDelay  SampleTime=-1
  veloc units : Gain  Gain=1/velocCanon  ParameterDataType=sfix(16)  ParameterScaling=2^0  OutDataType=sfix(16)  OutScaling=2^0  SaturateOnIntegerOverflow=on  OutDataTypeStr=Inherit: Same as input  ParamDataTypeStr=Inherit: Same as input
  displ : Outport  OutDataType=sfix(16)  OutScaling=2^0
  veloc : Outport  Port=2  OutDataType=sfix(16)  OutScaling=2^0
  tag scope: ch3a=global
  wires:
  friction/1(force) -> Sum/2  "friction force"
  veloc units/1 -> veloc/1
  Sum/1 -> div/1  "inertial force"
  force/1 -> Sum/1  "total force"
  mass/1 -> div/2
  double integrator/3(acc) -> term1/1
  div/1 -> double integrator/1(accel)
  double integrator/1(displ) -> displ/1, unit dly/1
  double integrator/2(veloc) -> veloc units/1, friction/1(veloc), unit dly1/1
  static force/1 -> Sum/5  "static force"
  damper/1 -> Sum/4  "damper force"
  unit dly1/1 -> damper/1
  [ch3b] -> Sum/3  "spring force"
  unit dly/1 -> [ch3a]

== system HybridControllerD3D3/model/ActuatorPayloadMdl/dynamic long channel #2/actuator/valve  model ==
  note: Auxiliary diagnostic output vector:
      | 1:   valve opening
      | 2:   C1 pressure
      | 3:   C2 pressure
      | 4:   delta pressure
      | 5:   force
      | 6:   velocity
      | 7:   C1 flow
      | 8:   C2 flow
      | 9:   total flow
      | 10: kinematic flow
      | 11: compressibility flow
      | 12: leakage flow
  note: Note: "1" and "2" denote actuator
      | cylinders on either side of the
      | actuator piston.  With positive
      | valve drive, oil is ported into
      | cylinder 1, resulting in positive
      | displacement.
  note: Parameter vector:
      | 1:   oil bulk modulus (force/displ^2)
      | 2:   servovalve delay (sec)
      | 3:   servovalve overlap
      | 4:   rated pressure (force/displ^2)
      | 5:   rated flow at rated pressure (displ^3/sec)
      | 6:   nominal flow at rated pressure (displ^3/sec)
      | 7:   actuator piston area 1 (displ^2)
      | 8:   actuator piston area 2 (displ^2)
      | 9:   actuator usable stroke 1 (displ)
      | 10: actuator usable stroke 2 (displ)
      | 11: actuator end cushion length 1 (displ)
      | 12: actuator end cushion length 2 (displ)
      | 13: actuator parasitic damping factor
      | 14: cross-chamber leakage factor (flow/press)
      | 15: ratio port openings according to area
      | 16: sample period (sec)
      |
      | Conversion factors used for converting
      | signals from external (user) to internal
      | (canonical) units:
      |
      | 17: displacement
      | 18: velocity
      | 19: force
      | 20: pressure
      | 21: flow
  cmd : Inport  OutDataType=sfix(16)  OutScaling=2^0
  displ : Inport  Port=2  OutDataType=sfix(16)  OutScaling=2^0
  veloc : Inport  Port=3  OutDataType=sfix(16)  OutScaling=2^0
  spl press : Inport  Port=4  OutDataType=sfix(16)  OutScaling=2^0
  rtn press : Inport  Port=5  OutDataType=sfix(16)  OutScaling=2^0
  abs : Abs  SaturateOnIntegerOverflow=on
  actuator : S-Function  FunctionName=actuator  Parameters=actParamsB  EnableBusSupport=off
  total flow sel : Selector  InputPortWidth=12  IndexOptions=Index vector (dialog)  Indices=9  OutputSizes=1
  force : Outport  OutDataType=sfix(16)  OutScaling=2^0
  flow : Outport  Port=2  OutDataType=sfix(16)  OutScaling=2^0
  wires:
  abs/1 -> flow/1
  actuator/2 -> total flow sel/1
  total flow sel/1 -> abs/1
  spl press/1 -> actuator/4
  rtn press/1 -> actuator/5
  cmd/1 -> actuator/1
  actuator/1 -> force/1
  displ/1 -> actuator/2
  veloc/1 -> actuator/3

== system HybridControllerD3D3/model/ActuatorPayloadMdl/dynamic long channel #2/payload ==
  force : Inport  OutDataType=sfix(16)  OutScaling=2^0
  Sum : Sum  Inputs=+----  OutDataType=sfix(16)  OutScaling=2^0  SaturateOnIntegerOverflow=on  InputSameDT=on  OutDataTypeStr=Inherit: Same as first input
  damper : Gain  Gain=damperB*damperCanon  ParameterDataType=sfix(16)  ParameterScaling=2^0  OutDataType=sfix(16)  OutScaling=2^0  SaturateOnIntegerOverflow=on  OutDataTypeStr=Inherit: Same as input  ParamDataTypeStr=Inherit: Same as input
  div : Product  Inputs=*/  OutDataType=sfix(16)  OutScaling=2^0  SaturateOnIntegerOverflow=on  InputSameDT=on  OutDataTypeStr=Inherit: Same as first input
  double integrator : Subsystem
  friction : Subsystem  mask{friction=frictionB*forceCanon, yieldDispl=yieldDisplB*lengthCanon, hysteresis=0}
      mask prompts: friction "Sliding friction"; yieldDispl "Equiv. yield displacement (in)"; hysteresis "Hysteresis constant"
  mass : Constant  Value=massB*massCanon  OutDataType=sfix(16)  OutScaling=2^0
  static force : Constant  Value=staticForceB*forceCanon  OutDataType=sfix(16)  OutScaling=2^0
  term1 : Terminator
  unit dly : UnitDelay  SampleTime=-1
  unit dly1 : UnitDelay  SampleTime=-1
  veloc units : Gain  Gain=1/velocCanon  ParameterDataType=sfix(16)  ParameterScaling=2^0  OutDataType=sfix(16)  OutScaling=2^0  SaturateOnIntegerOverflow=on  OutDataTypeStr=Inherit: Same as input  ParamDataTypeStr=Inherit: Same as input
  displ : Outport  OutDataType=sfix(16)  OutScaling=2^0
  veloc : Outport  Port=2  OutDataType=sfix(16)  OutScaling=2^0
  tag scope: ch4a=global
  wires:
  friction/1(force) -> Sum/2  "friction force"
  veloc units/1 -> veloc/1
  Sum/1 -> div/1  "inertial force"
  force/1 -> Sum/1  "total force"
  mass/1 -> div/2
  double integrator/3(acc) -> term1/1
  div/1 -> double integrator/1(accel)
  double integrator/1(displ) -> displ/1, unit dly/1
  double integrator/2(veloc) -> veloc units/1, friction/1(veloc), unit dly1/1
  static force/1 -> Sum/5  "static force"
  damper/1 -> Sum/4  "damper force"
  unit dly1/1 -> damper/1
  [ch4b] -> Sum/3  "spring force"
  unit dly/1 -> [ch4a]

== system HybridControllerD3D3/model/ActuatorPayloadMdl/dynamic short channel #1/actuator/valve  model ==
  note: Auxiliary diagnostic output vector:
      | 1:   valve opening
      | 2:   C1 pressure
      | 3:   C2 pressure
      | 4:   delta pressure
      | 5:   force
      | 6:   velocity
      | 7:   C1 flow
      | 8:   C2 flow
      | 9:   total flow
      | 10: kinematic flow
      | 11: compressibility flow
      | 12: leakage flow
  note: Note: "1" and "2" denote actuator
      | cylinders on either side of the
      | actuator piston.  With positive
      | valve drive, oil is ported into
      | cylinder 1, resulting in positive
      | displacement.
  note: Parameter vector:
      | 1:   oil bulk modulus (force/displ^2)
      | 2:   servovalve delay (sec)
      | 3:   servovalve overlap
      | 4:   rated pressure (force/displ^2)
      | 5:   rated flow at rated pressure (displ^3/sec)
      | 6:   nominal flow at rated pressure (displ^3/sec)
      | 7:   actuator piston area 1 (displ^2)
      | 8:   actuator piston area 2 (displ^2)
      | 9:   actuator usable stroke 1 (displ)
      | 10: actuator usable stroke 2 (displ)
      | 11: actuator end cushion length 1 (displ)
      | 12: actuator end cushion length 2 (displ)
      | 13: actuator parasitic damping factor
      | 14: cross-chamber leakage factor (flow/press)
      | 15: ratio port openings according to area
      | 16: sample period (sec)
      |
      | Conversion factors used for converting
      | signals from external (user) to internal
      | (canonical) units:
      |
      | 17: displacement
      | 18: velocity
      | 19: force
      | 20: pressure
      | 21: flow
  cmd : Inport  OutDataType=sfix(16)  OutScaling=2^0
  displ : Inport  Port=2  OutDataType=sfix(16)  OutScaling=2^0
  veloc : Inport  Port=3  OutDataType=sfix(16)  OutScaling=2^0
  spl press : Inport  Port=4  OutDataType=sfix(16)  OutScaling=2^0
  rtn press : Inport  Port=5  OutDataType=sfix(16)  OutScaling=2^0
  abs : Abs  SaturateOnIntegerOverflow=on
  actuator : S-Function  FunctionName=actuator  Parameters=actParamsA  EnableBusSupport=off
  total flow sel : Selector  InputPortWidth=12  IndexOptions=Index vector (dialog)  Indices=9  OutputSizes=1
  force : Outport  OutDataType=sfix(16)  OutScaling=2^0
  flow : Outport  Port=2  OutDataType=sfix(16)  OutScaling=2^0
  wires:
  abs/1 -> flow/1
  actuator/2 -> total flow sel/1
  total flow sel/1 -> abs/1
  spl press/1 -> actuator/4
  rtn press/1 -> actuator/5
  cmd/1 -> actuator/1
  actuator/1 -> force/1
  displ/1 -> actuator/2
  veloc/1 -> actuator/3

== system HybridControllerD3D3/model/ActuatorPayloadMdl/dynamic short channel #1/payload ==
  force : Inport  OutDataType=sfix(16)  OutScaling=2^0
  Sum : Sum  Inputs=+----  OutDataType=sfix(16)  OutScaling=2^0  SaturateOnIntegerOverflow=on  InputSameDT=on  OutDataTypeStr=Inherit: Same as first input
  damper : Gain  Gain=damperA*damperCanon  ParameterDataType=sfix(16)  ParameterScaling=2^0  OutDataType=sfix(16)  OutScaling=2^0  SaturateOnIntegerOverflow=on  OutDataTypeStr=Inherit: Same as input  ParamDataTypeStr=Inherit: Same as input
  div : Product  Inputs=*/  OutDataType=sfix(16)  OutScaling=2^0  SaturateOnIntegerOverflow=on  InputSameDT=on  OutDataTypeStr=Inherit: Same as first input
  double integrator : Subsystem
  friction : Subsystem  mask{friction=frictionA*forceCanon, yieldDispl=yieldDisplA*lengthCanon, hysteresis=0}
      mask prompts: friction "Sliding friction"; yieldDispl "Equiv. yield displacement (in)"; hysteresis "Hysteresis constant"
  mass : Constant  Value=massA*massCanon  OutDataType=sfix(16)  OutScaling=2^0
  static force : Constant  Value=staticForceA*forceCanon  OutDataType=sfix(16)  OutScaling=2^0
  term1 : Terminator
  unit dly : UnitDelay  SampleTime=-1
  unit dly1 : UnitDelay  SampleTime=-1
  veloc units : Gain  Gain=1/velocCanon  ParameterDataType=sfix(16)  ParameterScaling=2^0  OutDataType=sfix(16)  OutScaling=2^0  SaturateOnIntegerOverflow=on  OutDataTypeStr=Inherit: Same as input  ParamDataTypeStr=Inherit: Same as input
  displ : Outport  OutDataType=sfix(16)  OutScaling=2^0
  veloc : Outport  Port=2  OutDataType=sfix(16)  OutScaling=2^0
  tag scope: ch1a=global
  wires:
  friction/1(force) -> Sum/2  "friction force"
  veloc units/1 -> veloc/1
  Sum/1 -> div/1  "inertial force"
  force/1 -> Sum/1  "total force"
  mass/1 -> div/2
  double integrator/3(acc) -> term1/1
  div/1 -> double integrator/1(accel)
  double integrator/1(displ) -> displ/1, unit dly/1
  double integrator/2(veloc) -> veloc units/1, friction/1(veloc), unit dly1/1
  static force/1 -> Sum/5  "static force"
  damper/1 -> Sum/4  "damper force"
  unit dly1/1 -> damper/1
  [ch1b] -> Sum/3  "spring force"
  unit dly/1 -> [ch1a]

== system HybridControllerD3D3/model/ActuatorPayloadMdl/dynamic short channel #2/actuator/valve  model ==
  note: Auxiliary diagnostic output vector:
      | 1:   valve opening
      | 2:   C1 pressure
      | 3:   C2 pressure
      | 4:   delta pressure
      | 5:   force
      | 6:   velocity
      | 7:   C1 flow
      | 8:   C2 flow
      | 9:   total flow
      | 10: kinematic flow
      | 11: compressibility flow
      | 12: leakage flow
  note: Note: "1" and "2" denote actuator
      | cylinders on either side of the
      | actuator piston.  With positive
      | valve drive, oil is ported into
      | cylinder 1, resulting in positive
      | displacement.
  note: Parameter vector:
      | 1:   oil bulk modulus (force/displ^2)
      | 2:   servovalve delay (sec)
      | 3:   servovalve overlap
      | 4:   rated pressure (force/displ^2)
      | 5:   rated flow at rated pressure (displ^3/sec)
      | 6:   nominal flow at rated pressure (displ^3/sec)
      | 7:   actuator piston area 1 (displ^2)
      | 8:   actuator piston area 2 (displ^2)
      | 9:   actuator usable stroke 1 (displ)
      | 10: actuator usable stroke 2 (displ)
      | 11: actuator end cushion length 1 (displ)
      | 12: actuator end cushion length 2 (displ)
      | 13: actuator parasitic damping factor
      | 14: cross-chamber leakage factor (flow/press)
      | 15: ratio port openings according to area
      | 16: sample period (sec)
      |
      | Conversion factors used for converting
      | signals from external (user) to internal
      | (canonical) units:
      |
      | 17: displacement
      | 18: velocity
      | 19: force
      | 20: pressure
      | 21: flow
  cmd : Inport  OutDataType=sfix(16)  OutScaling=2^0
  displ : Inport  Port=2  OutDataType=sfix(16)  OutScaling=2^0
  veloc : Inport  Port=3  OutDataType=sfix(16)  OutScaling=2^0
  spl press : Inport  Port=4  OutDataType=sfix(16)  OutScaling=2^0
  rtn press : Inport  Port=5  OutDataType=sfix(16)  OutScaling=2^0
  abs : Abs  SaturateOnIntegerOverflow=on
  actuator : S-Function  FunctionName=actuator  Parameters=actParamsA  EnableBusSupport=off
  total flow sel : Selector  InputPortWidth=12  IndexOptions=Index vector (dialog)  Indices=9  OutputSizes=1
  force : Outport  OutDataType=sfix(16)  OutScaling=2^0
  flow : Outport  Port=2  OutDataType=sfix(16)  OutScaling=2^0
  wires:
  abs/1 -> flow/1
  actuator/2 -> total flow sel/1
  total flow sel/1 -> abs/1
  spl press/1 -> actuator/4
  rtn press/1 -> actuator/5
  cmd/1 -> actuator/1
  actuator/1 -> force/1
  displ/1 -> actuator/2
  veloc/1 -> actuator/3
